simulink model "Final_Project_1"  (R2023b)
settings: Solver=FixedStepAuto  StartTime=0.0  StopTime=inf  FixedStep=0.01  RelTol=1e-3  EnableMultiTasking=on
libraries: arduinolib x3, arduinosensorlib x1
settings Model: ExtModeTrigDuration=2  Creator=FM23  LastModifiedBy=FM23
settings OptimizationCC: EnhancedBackFolding=on  PassReuseOutputArgsAs=Individual arguments  ZeroExternalMemoryAtStartup=off  ZeroInternalMemoryAtStartup=off  MaxStackSize=64  OptimizeBlockOrder=speed  DifferentSizesBufferReuse=on  OptimizationCustomize=off  EfficientTunableParamExpr=on
settings DebuggingCC: ParameterTunabilityLossMsg=error
settings HardwareCC: ProdBitPerInt=16  ProdBitPerPointer=16  ProdBitPerSizeT=16  ProdBitPerPtrDiffT=16  ProdLargestAtomicFloat=None  ProdWordSize=8  ProdHWDeviceType=Atmel->AVR
settings SFSimCC: MATLABDynamicMemAlloc=off
settings RTWCC: Description=Embedded Coder  SystemTargetFile=ert.tlc  HardwareBoard=Arduino Mega 2560  TemplateMakefile=ert_default_tmf  Toolchain=Arduino AVR  BuildConfiguration=Faster Runs
settings CodeAppCC: ForceParamTrailComments=on  IgnoreCustomStorageClasses=off  OperatorAnnotations=on  SimulinkDataObjDesc=on  SFDataObjDesc=on  InsertBlockDesc=on
settings ERTTargetCC: SupportContinuousTime=on  SupportVariableSizeSignals=on  ExtModeTransport=3  ExtModeStaticAlloc=on  ExtModeAutomaticAllocSize=off  ExtModeStaticAllocSize=2048  ExtModeMexFile=ext_xcp  ExtModeIntrfLevel=Level2 - Open

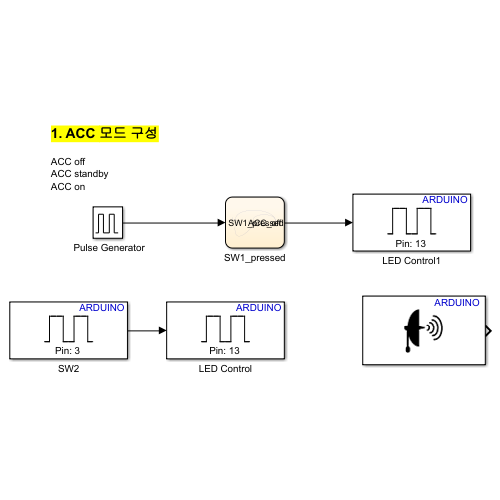
[thumbnail: Simulink's stored preview of the top-level diagram]
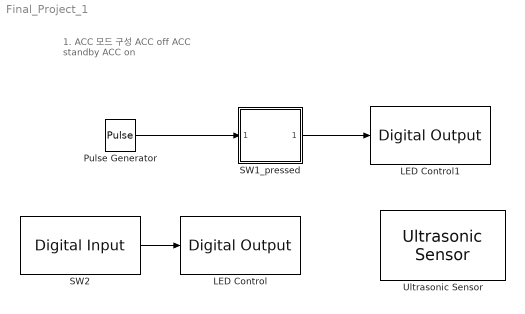
== system Final_Project_1 ==
  note: 1. ACC 모드 구성
      |
      | ACC off
      | ACC standby
      | ACC on
  " Pulse Generator" : DiscretePulseGenerator  PulseType=Time based  Period=3  PulseWidth=50
  LED Control : arduinolib/Digital Output  pinNumber=13  Direction=output  blockPlatform=arduino
  LED Control1 : arduinolib/Digital Output  pinNumber=13  Direction=output  blockPlatform=arduino
  SW1_pressed : Stateflow chart  TreatAsAtomicUnit=on
  SW2 : arduinolib/Digital Input  pinNumber=3  mode=Default  Direction=input  SampleTime=-1  blockPlatform=arduino
  Ultrasonic Sensor : arduinosensorlib/Ultrasonic Sensor  NumSignalPins=1  TrigPin=4  EchoPin=5  SignalPin=3  SampleTime_=0.1  blockPlatform=ARDUINO
  wires:
  " Pulse Generator"/1 -> SW1_pressed/1(SW1_pressed)
  SW2/1 -> LED Control/1
  SW1_pressed/1(" ACC_off") -> LED Control1/1

== stateflow chart Final_Project_1/SW1_pressed ==
  state ACC_off
    settings: description=LED_OFF();
  state ACC_standby
    settings: description=LED_FLASH(0.2);
  state ACC_on
    settings: description=LED_ON();
  ACC_on -> ACC_off : [SW1_pressed]
  ACC_standby -> ACC_on : [SW1_pressed]
  (default) -> ACC_off
  ACC_off -> ACC_standby : [SW1_pressed]
  data: ACC_off output boolean; SW1_pressed input
